simulink model "L0206"  (Simulink 9.1)
settings: Solver=VariableStepAuto  StartTime=0.0  StopTime=10.0  RelTol=1e-3
libraries: simulink x4
settings Model: Creator=Asus  LastModifiedBy=Asus
settings DataIOCC: SaveFormat=Dataset
settings OptimizationCC: LifeSpan=auto
settings DebuggingCC: UnderspecifiedInitializationDetection=Simplified  MergeDetectMultiDrivingBlocksExec=error  SFUnexpectedBacktrackingDiag=error  SFNoUnconditionalDefaultTransitionDiag=error  SFExecutionAtInitializationDiag=warning
settings HardwareCC: ProdBitPerPointer=64  ProdBitPerSizeT=64  ProdBitPerPtrDiffT=64  ProdLargestAtomicFloat=Float  ProdIntDivRoundTo=Zero  ProdEndianess=LittleEndian  ProdWordSize=64  ProdHWDeviceType=Intel->x86-64 (Windows64)
settings ModelReferenceCC: PropagateSignalLabelsOutOfModel=on
settings CodeAppCC: StateflowObjectComments=off
settings GRTTargetCC: TargetLangStandard=C99 (ISO)  CombineOutputUpdateFcns=on  GRTInterface=off
settings ConfigComp: CovMetricSettings=dwe  CovHtmlReporting=off  CovSaveCumulativeToWorkspaceVar=off  CovSaveSingleToWorkspaceVar=off  CovExternalEMLEnable=on

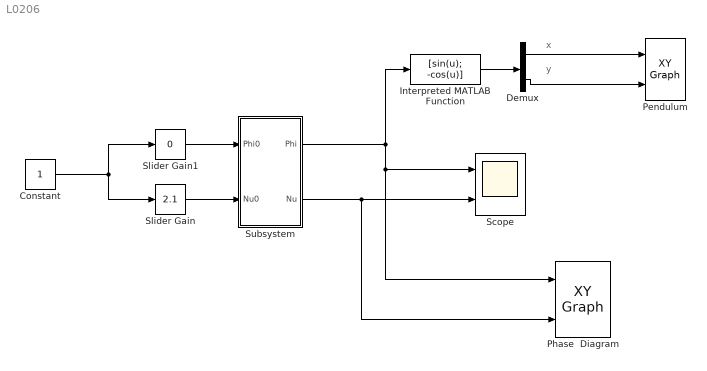
== system L0206 ==
  note: y
  note: x
  Constant : Constant
  Demux : Demux  Outputs=2
  Interpreted MATLAB Function : MATLABFcn  MATLABFcn=[sin(u); -cos(u)]  OutputDimensions=2
  "Pendulum " : simulink/Sinks/XY Graph  xmin=-1  xmax=1  ymin=-1  ymax=1  st=-1
  "Phase  Diagram " : simulink/Sinks/XY Graph  xmin=-1  xmax=1  ymin=-1  ymax=1  st=-1
  Scope : Scope  NumInputPorts=2
  Slider Gain : simulink/Math Operations/Slider Gain  gain=2.1  low=0  high=5
  Slider Gain1 : simulink/Math Operations/Slider Gain  gain=0  low=0  high=1
  Subsystem : Subsystem
  wires:
  Demux/1 -> "Pendulum "/1
  Demux/2 -> "Pendulum "/2
  Interpreted MATLAB Function/1 -> Demux/1
  Subsystem/1("Phi ") -> Scope/1, "Phase  Diagram "/1, Interpreted MATLAB Function/1
  Subsystem/2(Nu) -> Scope/2, "Phase  Diagram "/2
  Constant/1 -> Slider Gain/1, Slider Gain1/1
  Slider Gain1/1 -> Subsystem/1("Phi0 ")
  Slider Gain/1 -> Subsystem/2(Nu0)

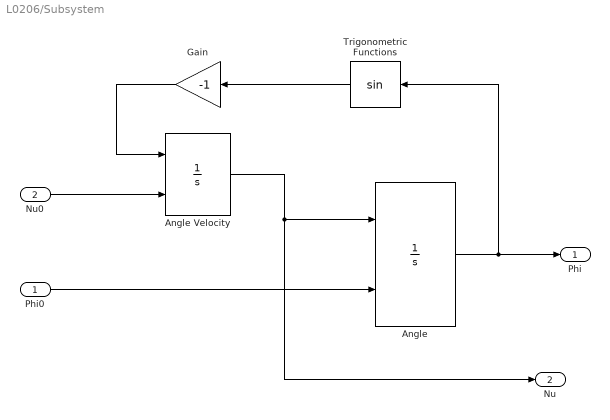
== system L0206/Subsystem ==
  "Phi0 " : Inport
  Nu0 : Inport  Port=2
  Angle : Integrator  InitialConditionSource=external
  Angle Velocity : Integrator  InitialConditionSource=external
  Gain : Gain  Gain=-1
  Trigonometric Functions : Trigonometry
  "Phi " : Outport
  Nu : Outport  Port=2
  wires:
  Nu0/1 -> Angle Velocity/2
  Gain/1 -> Angle Velocity/1
  Angle Velocity/1 -> Nu/1, Angle/1
  "Phi0 "/1 -> Angle/2
  Angle/1 -> Trigonometric Functions/1, "Phi "/1
  Trigonometric Functions/1 -> Gain/1
